simulink model "Aufgabe_5_2_5_Vereinfachte_Drehtellersteuerung"  (R2023b)
settings: Solver=ode3  StartTime=0.0  StopTime=40  FixedStep=0.01  RelTol=1e-3  EnableMultiTasking=on
values from neighbouring files (symbols this model uses):
  A = 5    [Aufgabe_4_3_3_Parameter_Drehtellers.m]
  I = 0.5    [Aufgabe_4_3_3_Parameter_Drehtellers.m]
  igetr = 1080    [Aufgabe_4_3_3_Parameter_Drehtellers.m]
  K = 8    [Aufgabe_4_3_3_Parameter_Drehtellers.m]
  MRK = 1    [Aufgabe_4_3_3_Parameter_Drehtellers.m]
  PHI = 0.001    [Aufgabe_4_3_3_Parameter_Drehtellers.m]
  Ra = 40    [Aufgabe_4_3_3_Parameter_Drehtellers.m]
  U = 24    [Aufgabe_4_3_3_Parameter_Drehtellers.m]
settings Model: Creator=JCP  LastModifiedBy=JCP

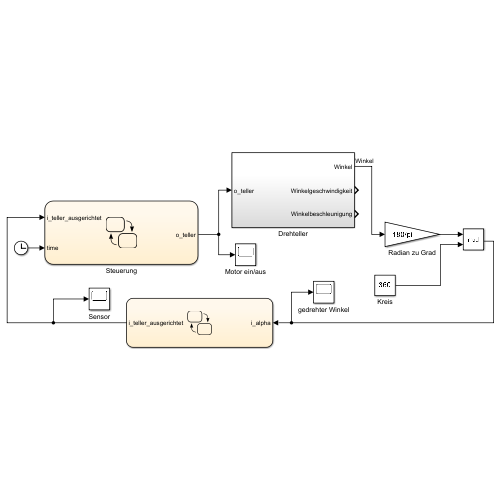
[thumbnail: Simulink's stored preview of the top-level diagram]
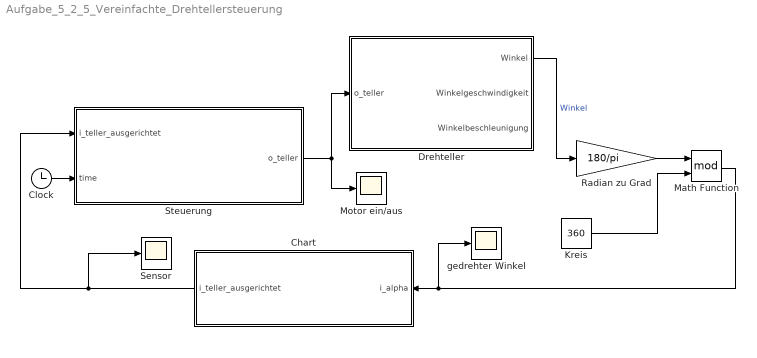
== system Aufgabe_5_2_5_Vereinfachte_Drehtellersteuerung ==
  Chart : Stateflow chart  TreatAsAtomicUnit=on
  Clock : Clock
  Drehteller : Subsystem
  Kreis : Constant  Value=360
  Math Function : Math  Operator=mod  SignedPower=on
  Motor ein/aus : Scope
  Radian zu Grad : Gain  Gain=180/pi
  Sensor : Scope
  Steuerung : Stateflow chart  TreatAsAtomicUnit=on
  gedrehter Winkel : Scope
  wires:
  Math Function/1 -> Chart/1(i_alpha), gedrehter Winkel/1
  Steuerung/1(o_teller) -> Drehteller/1(o_teller), Motor ein/aus/1
  Chart/1(i_teller_ausgerichtet) -> Steuerung/1(i_teller_ausgerichtet), Sensor/1
  Clock/1 -> Steuerung/2(time)
  Radian zu Grad/1 -> Math Function/1
  Kreis/1 -> Math Function/2
  Drehteller/1(Winkel) -> Radian zu Grad/1  "Winkel"

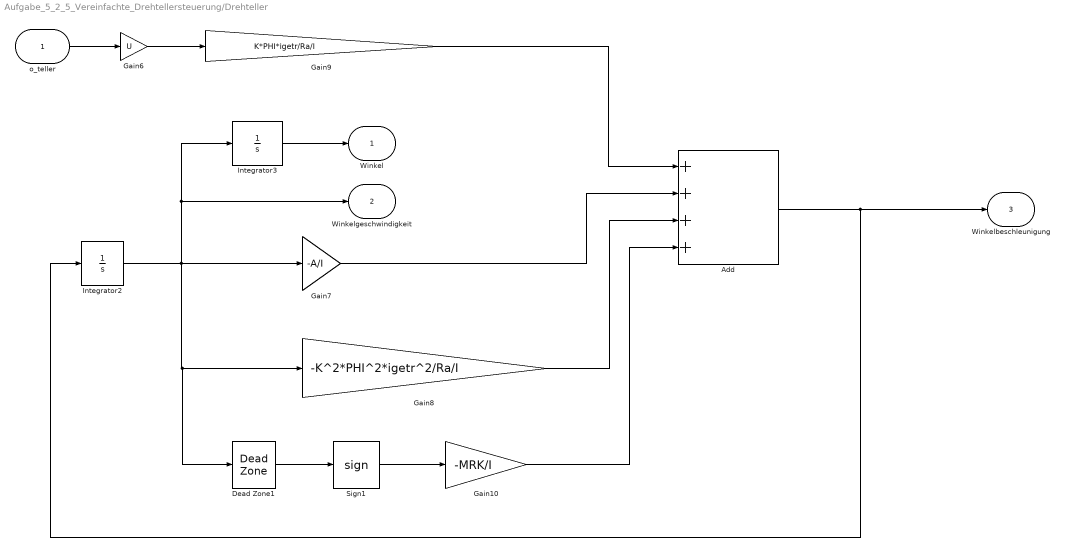
== system Aufgabe_5_2_5_Vereinfachte_Drehtellersteuerung/Drehteller ==
  o_teller : Inport
  Add : Sum  Inputs=++++
  Dead Zone1 : DeadZone
  Gain10 : Gain  Gain=-MRK/I
  Gain6 : Gain  Gain=U
  Gain7 : Gain  Gain=-A/I
  Gain8 : Gain  Gain=-K^2*PHI^2*igetr^2/Ra/I
  Gain9 : Gain  Gain=K*PHI*igetr/Ra/I
  Integrator2 : Integrator
  Integrator3 : Integrator
  Sign1 : Signum
  Winkel : Outport
  Winkelgeschwindigkeit : Outport  Port=2
  Winkelbeschleunigung : Outport  Port=3
  wires:
  Gain6/1 -> Gain9/1
  Sign1/1 -> Gain10/1
  Gain7/1 -> Add/2
  Gain10/1 -> Add/4
  Gain8/1 -> Add/3
  Integrator3/1 -> Winkel/1
  Integrator2/1 -> Winkelgeschwindigkeit/1, Integrator3/1, Dead Zone1/1, Gain8/1, Gain7/1
  Gain9/1 -> Add/1
  Dead Zone1/1 -> Sign1/1
  o_teller/1 -> Gain6/1
  Add/1 -> Integrator2/1, Winkelbeschleunigung/1

== stateflow chart Aufgabe_5_2_5_Vereinfachte_Drehtellersteuerung/Steuerung ==
  state Wait
    entry: start_time =  time;
  state Drehen
    entry: o_teller = 1
  state Sensorabfrage
    exit: o_teller = 0
  (default) -> Wait
  Wait -> Drehen : [time - 2 >= start_time]
  Sensorabfrage -> Wait : [i_teller_ausgerichtet == 1 ]
  Drehen -> Sensorabfrage : after(0.5,sec)
  data: o_teller output double; i_teller_ausgerichtet input; time input; start_time local double

== stateflow chart Aufgabe_5_2_5_Vereinfachte_Drehtellersteuerung/Chart ==
  state Winkelsensor
    state Ausgerichtet
      entry: i_teller_ausgerichtet = 1;
    state Nicht_ausgerichtet
      entry: i_teller_ausgerichtet = 0;
    Nicht_ausgerichtet -> Ausgerichtet : [mod(i_alpha, 90) >88 || mod(i_alpha, 90) < 2]
    (default) -> Nicht_ausgerichtet
    Ausgerichtet -> Nicht_ausgerichtet : [mod(i_alpha, 90) >= 2 && mod(i_alpha, 90) <= 88]
  data: i_alpha input; i_teller_ausgerichtet output
